simulink model "simulink_template_1_1"  (R2025b)
settings: Solver=ode4  StartTime=0.0  StopTime=T_SIMULATION  FixedStep=0.001  RelTol=1e-3
values from neighbouring files (symbols this model uses):
  d = 0.165    [live_script.m]    (also in script_1_1.m; script_1_simulation.m; script_2_motion_planning.m)
  OMEGA_L = 10    [live_script.m]    (also in script_1_1.m; script_1_simulation.m)
  OMEGA_R = -10    [live_script.m]    (also in script_1_1.m; script_1_simulation.m)
  Q_INITIAL = [1;1;0]    [live_script.m]    (also in script_1_1.m = [0;0;0]; script_1_simulation.m)
  r = 0.03    [live_script.m]    (also in script_1_1.m; script_1_simulation.m; script_2_motion_planning.m)
settings Model: Creator=alber  LastModifiedBy=llp

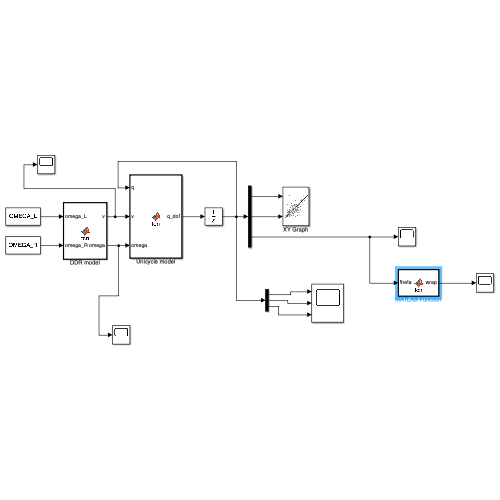
[thumbnail: Simulink's stored preview of the top-level diagram]
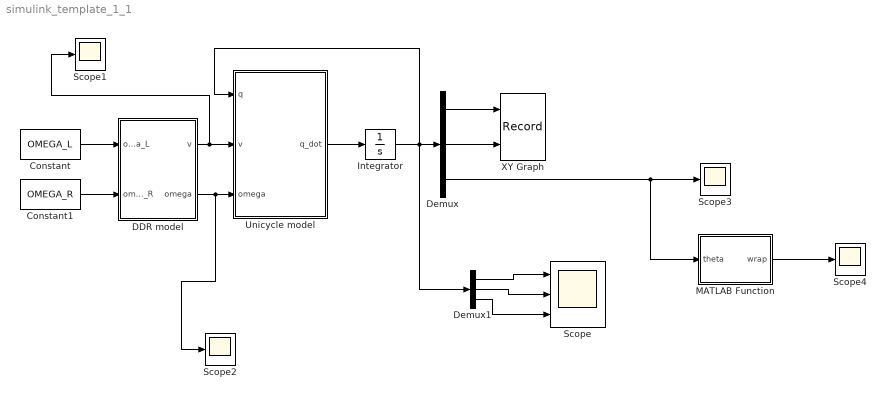
== system simulink_template_1_1 ==
  Constant : Constant  Value=OMEGA_L
  Constant1 : Constant  Value=OMEGA_R
  DDR model : MATLAB Function  TreatAsAtomicUnit=on
  Demux : Demux  Outputs=3
  Demux1 : Demux  Outputs=3
  Integrator : Integrator  InitialCondition=Q_INITIAL
  MATLAB Function : MATLAB Function  TreatAsAtomicUnit=on
  Scope : Scope  NumInputPorts=3
      settings: ActiveDisplayYMinimum=-18.558005528495297  ActiveDisplayYMaximum=3.3856861200938342
  Scope{1..4} (4 alike) : Scope
      Scope1 settings: ActiveDisplayYMinimum=-1  ActiveDisplayYMaximum=1
      Scope2 settings: ActiveDisplayYMinimum=-1  ActiveDisplayYMaximum=1  DataLoggingVariableName=ScopeData2
      Scope3 settings: ActiveDisplayYMinimum=-40.909090909088462  ActiveDisplayYMaximum=4.5454545454542723  DataLoggingVariableName=ScopeData3
      Scope4 settings: DataLoggingVariableName=ScopeData4
  Unicycle model : MATLAB Function  TreatAsAtomicUnit=on
  XY Graph : Record  NumPorts=2.0  FileSettingsInternal="{\"entries\":[{\"content\":{\"excelSettings\":{\"content\":{},\"type\":\"Streamout.ExcelSettings\"},\"parquetSettings\":{\"content\":{},\"type\":\"Streamout.ParquetSettings\"}},\"type\":\"Streamout.FileSettingStorage\",\"uuid\":\"\"}],\"packageUris\":[\"http:\\/\\/schema.mathworks.com\\/mf0\\/streamout_blocks\\/R2020a\"],\"version\":\"1.0\"}"  FrameSettings=[0, 0]  Layout=[1 1]  SignalsInternal="{\"entries\":[{\"content\":{\"signals\":[{\"content\":{\"blockPath\":[],\"dimensions\":[1,1],\"domain\":\"\",\"lineColor\":\"#a2142f\",\"plots\":[ 1 ],\"port\":1,\"sid\":[\"\"],\"signalID\":1,\"signalName\":\"Demux:1\"},\"type\":\"RecordBlkView.Signal\",\"uuid\":\"\"},{\"content\":{\"blockPath\":[],\"dimensions\":[1,1],\"domain\":\"\",\"lineColor\":\"#139fff\",\"plots\":[ 1 ],\"port\":2,\"sid\":[\"\"],\"signalID\":2,\"signalName\":\"Demux:2\"},\"type\":\"RecordBlkView.Signal\",\"uuid\":\"\"}]},\"type\":\"RecordBlkView.InputSignals\",\"uuid\":\"\"}],\"packageUris\":[\"http:\\/\\/schema.mathworks.com\\/mf0\\/streamout_blocks\\/R2020a\"],\"version\":\"1.0\"}"  VisualizationBindings="{\"xyplotplugin\":{\"info\":[{\"series\":[{\"bindingParametersList\":[{\"parameter\":\"X-Axis\",\"signalID\":1,\"signalName\":\"Demux:1\"},{\"parameter\":\"Y-Axis\",\"signalID\":2,\"signalName\":\"Demux:2\"},{\"parameter\":\"X-Axis\",\"signalID\":1,\"signalName\":\"Demux:1\"},{\"parameter\":\"Y-Axis\",\"signalID\":2,\"signalName\":\"Demux:2\"}],\"seriesID\":0}],\"subplotID\":1}]}}"  CompatibilityTag=XY
  wires:
  Constant/1 -> DDR model/1(omega_L)
  Unicycle model/1(q_dot) -> Integrator/1
  DDR model/2(omega) -> Scope2/1, Unicycle model/3(omega)
  DDR model/1(v) -> Scope1/1, Unicycle model/2(v)
  Integrator/1 -> Demux1/1, Demux/1, Unicycle model/1(q)
  Demux/2 -> XY Graph/2
  Demux/1 -> XY Graph/1
  Constant1/1 -> DDR model/2(omega_R)
  Demux1/1 -> Scope/1
  Demux1/2 -> Scope/2
  Demux1/3 -> Scope/3
  Demux/3 -> MATLAB Function/1(theta), Scope3/1
  MATLAB Function/1(wrap) -> Scope4/1

== matlab function simulink_template_1_1/Unicycle model ==
  data: q input; v input; q_dot output; omega input; r parameter; d parameter
function q_dot = fcn(q, v, omega, r, d)
%write the unicycle model
q_dot= zeros(3,1);

q_dot(1) = v*cos(q(3));
q_dot(2) = v*sin(q(3));
q_dot(3) = omega;

== matlab function simulink_template_1_1/DDR model ==
  data: omega_L input; v output; omega_R input; omega output; r parameter; d parameter
function [v, omega] = fcn(omega_L, omega_R, r, d)
%write the DDR model and return v and omega
v=r*(omega_L+omega_R)/2;
omega=r*(omega_R-omega_L)/d;

== matlab function simulink_template_1_1/MATLAB Function ==
  data: theta input; wrap output
function wrap = fcn(theta)

wrap = mod(theta+pi,2*pi)-pi ;
